simulink model "gm_lab3_p9"  (R2020a)
settings: Solver=VariableStepAuto  StartTime=0.0  StopTime=mp.test_signal.duration  RelTol=1e-3
InitFcn:
  | sm_callback_init
StopFcn:
  | sm_callback_stop
undefined symbols (not defined in the file or in its folder): mp
libraries: hdlsllib x10, simulink x3
(part 1 of 2)
settings Model: Creator=Owner  LastModifiedBy=Owner
settings DataIOCC: ReturnWorkspaceOutputs=off
settings OptimizationCC: BlockReduction=off  ConditionallyExecuteInputs=off  DefaultParameterBehavior=Inlined
settings DebuggingCC: AlgebraicLoopMsg=error  ArtificialAlgebraicLoopMsg=none  InheritedTsInSrcMsg=none
settings HardwareCC: ProdBitPerPointer=32  ProdBitPerSizeT=32  ProdBitPerPtrDiffT=32  ProdLargestAtomicFloat=None  ProdIntDivRoundTo=Undefined  ProdEndianess=Unspecified  ProdWordSize=32  ProdHWDeviceType=ASIC/FPGA->ASIC/FPGA  TargetBitPerPointer=64  TargetBitPerSizeT=64  TargetBitPerPtrDiffT=64  TargetLongLongMode=on  TargetIntDivRoundTo=Zero  TargetEndianess=LittleEndian  TargetWordSize=64  TargetHWDeviceType=Custom Processor->MATLAB Host Computer  ProdEqTarget=off

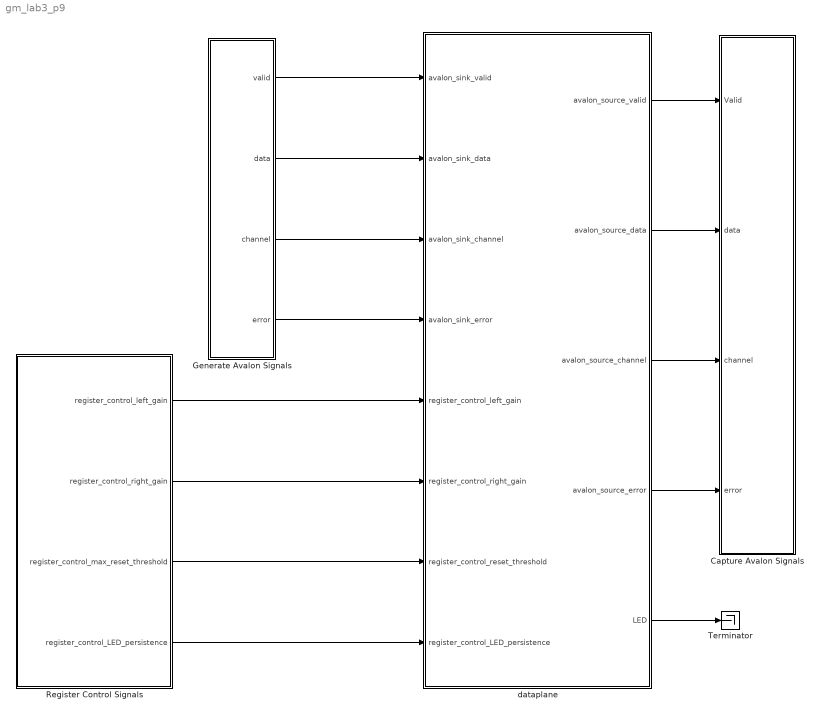
== system gm_lab3_p9 ==
  Capture Avalon Signals : Subsystem
  Generate Avalon Signals : Subsystem
  Register Control Signals : Subsystem
  Terminator : Terminator
  dataplane : Subsystem  TreatAsAtomicUnit=on
  wires:
  dataplane/5(LED) -> Terminator/1
  Register Control Signals/4(register_control_LED_persistence) -> dataplane/8(register_control_LED_persistence)
  Register Control Signals/3(register_control_max_reset_threshold) -> dataplane/7(register_control_reset_threshold)
  Register Control Signals/1(register_control_left_gain) -> dataplane/5(register_control_left_gain)
  Register Control Signals/2(register_control_right_gain) -> dataplane/6(register_control_right_gain)
  dataplane/4(avalon_source_error) -> Capture Avalon Signals/4(error)
  dataplane/3(avalon_source_channel) -> Capture Avalon Signals/3(channel)
  dataplane/2(avalon_source_data) -> Capture Avalon Signals/2(data)
  dataplane/1(avalon_source_valid) -> Capture Avalon Signals/1(Valid)
  Generate Avalon Signals/4(error) -> dataplane/4(avalon_sink_error)
  Generate Avalon Signals/3(channel) -> dataplane/3(avalon_sink_channel)
  Generate Avalon Signals/2(data) -> dataplane/2(avalon_sink_data)
  Generate Avalon Signals/1(valid) -> dataplane/1(avalon_sink_valid)

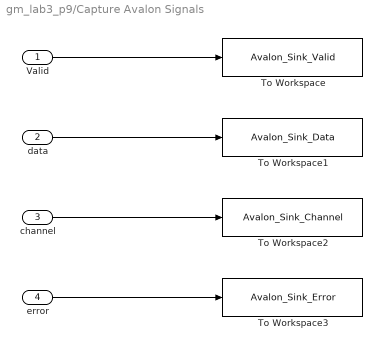
== system gm_lab3_p9/Capture Avalon Signals ==
  Valid : Inport
  data : Inport  Port=2
  channel : Inport  Port=3
  error : Inport  Port=4
  To Workspace : ToWorkspace  VariableName=Avalon_Sink_Valid  SampleTime=-1
      settings: Save2DSignal=2-D array (concatenate along first dimension)
  To Workspace1 : ToWorkspace  VariableName=Avalon_Sink_Data  SampleTime=-1
      settings: Save2DSignal=2-D array (concatenate along first dimension)
  To Workspace2 : ToWorkspace  VariableName=Avalon_Sink_Channel  SampleTime=-1
      settings: Save2DSignal=2-D array (concatenate along first dimension)
  To Workspace3 : ToWorkspace  VariableName=Avalon_Sink_Error  SampleTime=-1
      settings: Save2DSignal=2-D array (concatenate along first dimension)
  wires:
  error/1 -> To Workspace3/1
  channel/1 -> To Workspace2/1
  data/1 -> To Workspace1/1
  Valid/1 -> To Workspace/1

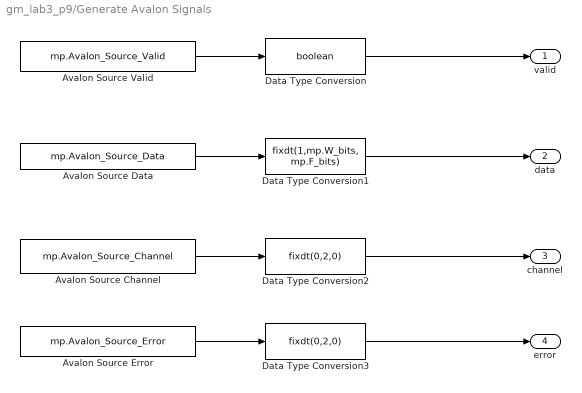
== system gm_lab3_p9/Generate Avalon Signals ==
  Avalon Source Channel : FromWorkspace  VariableName=mp.Avalon_Source_Channel  OutDataTypeStr=double  SampleTime=mp.Ts_system
  Avalon Source Data : FromWorkspace  VariableName=mp.Avalon_Source_Data  OutDataTypeStr=double  SampleTime=mp.Ts_system
  Avalon Source Error : FromWorkspace  VariableName=mp.Avalon_Source_Error  OutDataTypeStr=double  SampleTime=mp.Ts_system
  Avalon Source Valid : FromWorkspace  VariableName=mp.Avalon_Source_Valid  OutDataTypeStr=double  SampleTime=mp.Ts_system
  Data Type Conversion : DataTypeConversion  OutDataTypeStr=boolean  RndMeth=Nearest
  Data Type Conversion1 : DataTypeConversion  OutDataTypeStr=fixdt(1,mp.W_bits, mp.F_bits)  RndMeth=Nearest
  Data Type Conversion2 : DataTypeConversion  OutDataTypeStr=fixdt(0,2,0)  RndMeth=Nearest
  Data Type Conversion3 : DataTypeConversion  OutDataTypeStr=fixdt(0,2,0)  RndMeth=Nearest
  valid : Outport
  data : Outport  Port=2
  channel : Outport  Port=3
  error : Outport  Port=4
  wires:
  Avalon Source Error/1 -> Data Type Conversion3/1
  Data Type Conversion3/1 -> error/1
  Avalon Source Channel/1 -> Data Type Conversion2/1
  Data Type Conversion2/1 -> channel/1
  Data Type Conversion1/1 -> data/1
  Avalon Source Data/1 -> Data Type Conversion1/1
  Avalon Source Valid/1 -> Data Type Conversion/1
  Data Type Conversion/1 -> valid/1

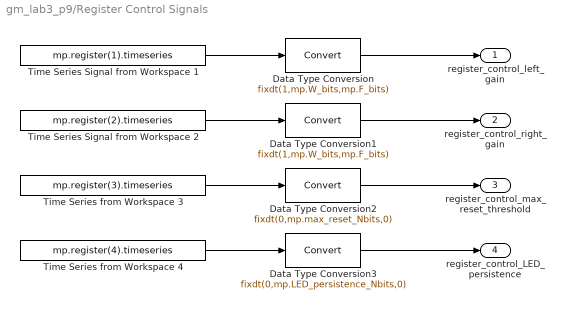
== system gm_lab3_p9/Register Control Signals ==
  Data Type Conversion : DataTypeConversion  OutDataTypeStr=fixdt(1,mp.W_bits,mp.F_bits)
  Data Type Conversion1 : DataTypeConversion  OutDataTypeStr=fixdt(1,mp.W_bits,mp.F_bits)
  Data Type Conversion2 : DataTypeConversion  OutDataTypeStr=fixdt(0,mp.max_reset_Nbits,0)
  Data Type Conversion3 : DataTypeConversion  OutDataTypeStr=fixdt(0,mp.LED_persistence_Nbits,0)
  Time Series Signal from Workspace 1 : FromWorkspace  VariableName=mp.register(1).timeseries  OutDataTypeStr=double  SampleTime=mp.Ts_system
  Time Series Signal from Workspace 2 : FromWorkspace  VariableName=mp.register(2).timeseries  OutDataTypeStr=double  SampleTime=mp.Ts_system
  Time Series from Workspace 3 : FromWorkspace  VariableName=mp.register(3).timeseries  OutDataTypeStr=double  SampleTime=mp.Ts_system
  Time Series from Workspace 4 : FromWorkspace  VariableName=mp.register(4).timeseries  OutDataTypeStr=double  SampleTime=mp.Ts_system
  register_control_left_gain : Outport
  register_control_right_gain : Outport  Port=2
  register_control_max_reset_threshold : Outport  Port=3
  register_control_LED_persistence : Outport  Port=4
  wires:
  Time Series from Workspace 3/1 -> Data Type Conversion2/1
  Time Series from Workspace 4/1 -> Data Type Conversion3/1
  Data Type Conversion3/1 -> register_control_LED_persistence/1
  Data Type Conversion2/1 -> register_control_max_reset_threshold/1
  Data Type Conversion1/1 -> register_control_right_gain/1
  Time Series Signal from Workspace 2/1 -> Data Type Conversion1/1
  Data Type Conversion/1 -> register_control_left_gain/1
  Time Series Signal from Workspace 1/1 -> Data Type Conversion/1

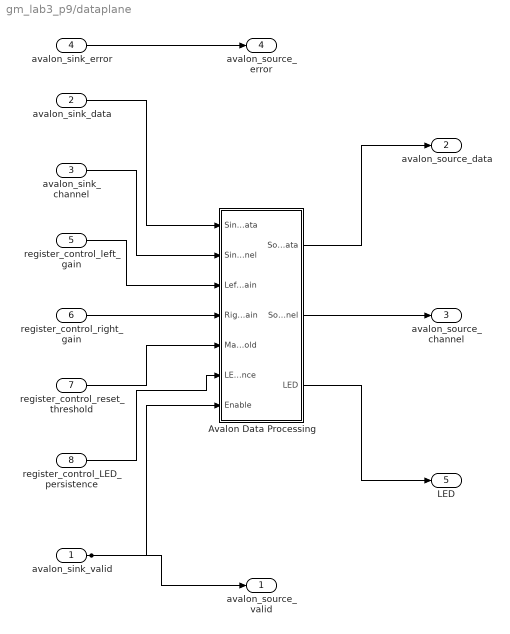
== system gm_lab3_p9/dataplane ==
  avalon_sink_valid : Inport  OutDataTypeStr=boolean  PortDimensions=1  SampleTime=1.01725260416667e-08
  avalon_sink_data : Inport  Port=2  OutDataTypeStr=fixdt(1, 32, 28)  PortDimensions=1  SampleTime=1.01725260416667e-08
  avalon_sink_channel : Inport  Port=3  OutDataTypeStr=fixdt(0, 2, 0)  PortDimensions=1  SampleTime=1.01725260416667e-08
  avalon_sink_error : Inport  Port=4  OutDataTypeStr=fixdt(0, 2, 0)  PortDimensions=1  SampleTime=1.01725260416667e-08
  register_control_left_gain : Inport  Port=5  OutDataTypeStr=fixdt(1, 32, 28)  PortDimensions=1  SampleTime=1.01725260416667e-08
  register_control_right_gain : Inport  Port=6  OutDataTypeStr=fixdt(1, 32, 28)  PortDimensions=1  SampleTime=1.01725260416667e-08
  register_control_reset_threshold : Inport  Port=7  OutDataTypeStr=fixdt(0, 18, 0)  PortDimensions=1  SampleTime=1.01725260416667e-08
  register_control_LED_persistence : Inport  Port=8  OutDataTypeStr=fixdt(0, 15, 0)  PortDimensions=1  SampleTime=1.01725260416667e-08
  Avalon Data Processing : Subsystem
  avalon_source_valid : Outport  VectorParamsAs1DForOutWhenUnconnected=off
  avalon_source_data : Outport  Port=2  VectorParamsAs1DForOutWhenUnconnected=off
  avalon_source_channel : Outport  Port=3  VectorParamsAs1DForOutWhenUnconnected=off
  avalon_source_error : Outport  Port=4  VectorParamsAs1DForOutWhenUnconnected=off
  LED : Outport  Port=5  VectorParamsAs1DForOutWhenUnconnected=off
  wires:
  avalon_sink_valid/1 -> avalon_source_valid/1, Avalon Data Processing/7(Enable)
  avalon_sink_data/1 -> Avalon Data Processing/1(Sink_Data)
  avalon_sink_channel/1 -> Avalon Data Processing/2(Sink_Channel)
  avalon_sink_error/1 -> avalon_source_error/1
  register_control_left_gain/1 -> Avalon Data Processing/3(Left_Gain)
  register_control_right_gain/1 -> Avalon Data Processing/4(Right_Gain)
  register_control_reset_threshold/1 -> Avalon Data Processing/5(Max_Reset_Threshold)
  register_control_LED_persistence/1 -> Avalon Data Processing/6(LED_persistence)
  Avalon Data Processing/1(Source_Data) -> avalon_source_data/1
  Avalon Data Processing/2(Source_Channel) -> avalon_source_channel/1
  Avalon Data Processing/3(LED) -> LED/1

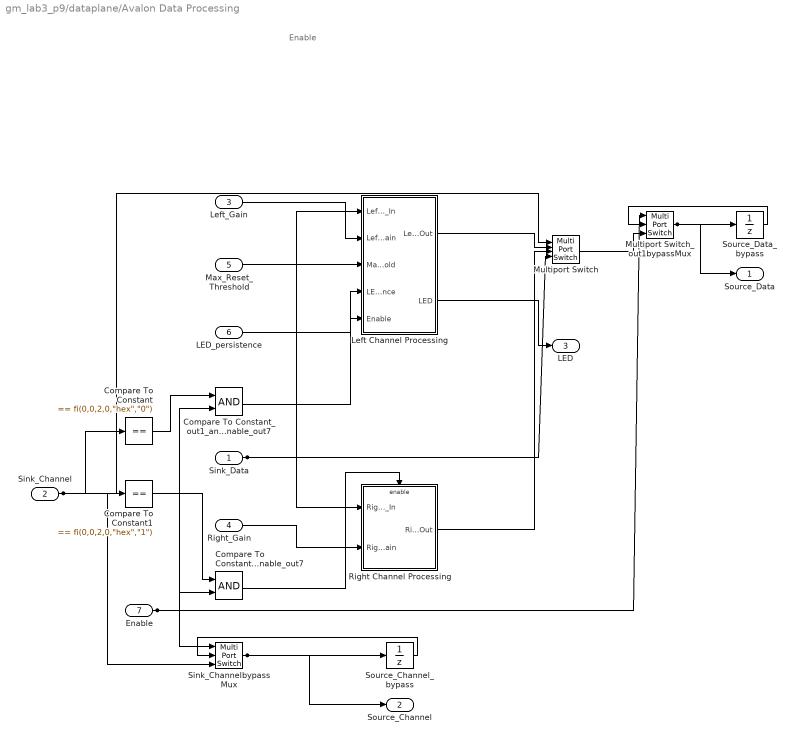
== system gm_lab3_p9/dataplane/Avalon Data Processing ==
  note: Enable
  Sink_Data : Inport  OutDataTypeStr=fixdt(1, 32, 28)  PortDimensions=1  SampleTime=1.01725260416667e-08
  Sink_Channel : Inport  Port=2  OutDataTypeStr=fixdt(0, 2, 0)  PortDimensions=1  SampleTime=1.01725260416667e-08
  Left_Gain : Inport  Port=3  OutDataTypeStr=fixdt(1, 32, 28)  PortDimensions=1  SampleTime=1.01725260416667e-08
  Right_Gain : Inport  Port=4  OutDataTypeStr=fixdt(1, 32, 28)  PortDimensions=1  SampleTime=1.01725260416667e-08
  Max_Reset_Threshold : Inport  Port=5  OutDataTypeStr=fixdt(0, 18, 0)  PortDimensions=1  SampleTime=1.01725260416667e-08
  LED_persistence : Inport  Port=6  OutDataTypeStr=fixdt(0, 15, 0)  PortDimensions=1  SampleTime=1.01725260416667e-08
  Enable : Inport  Port=7  OutDataTypeStr=boolean  SampleTime=1.01725260416667e-08
  Compare To Constant : simulink/Logic and Bit Operations/Compare To Constant  relop===  const="fi(0,0,2,0,\"hex\",\"0\")"  OutDataTypeStr=boolean
  Compare To Constant1 : simulink/Logic and Bit Operations/Compare To Constant  relop===  const="fi(0,0,2,0,\"hex\",\"1\")"  OutDataTypeStr=boolean
  Compare To Constant1_out1_and_Enable_out7 : Logic  AllPortsSameDT=off  OutDataTypeStr=boolean  SampleTime=1.01725260416667e-08
  Compare To Constant_out1_and_Enable_out7 : Logic  AllPortsSameDT=off  OutDataTypeStr=boolean  SampleTime=1.01725260416667e-08
  Left Channel Processing : Subsystem
  Multiport Switch : MultiPortSwitch  DataPortOrder=Zero-based contiguous  DiagnosticForDefault=None  zeroidx=on  OutDataTypeStr=fixdt(1, 32, 28)  SampleTime=1.01725260416667e-08
  Multiport Switch_out1bypassMux : MultiPortSwitch  DataPortOrder=Zero-based contiguous  Inputs=2  zeroidx=on  OutDataTypeStr=fixdt(1, 32, 28)  SampleTime=1.01725260416667e-08
  Right Channel Processing : Subsystem
  Sink_ChannelbypassMux : MultiPortSwitch  DataPortOrder=Zero-based contiguous  Inputs=2  zeroidx=on  OutDataTypeStr=fixdt(0, 2, 0)  SampleTime=1.01725260416667e-08
  Source_Channel_bypass : UnitDelay  SampleTime=1.01725260416667e-08
  Source_Data_bypass : UnitDelay  SampleTime=1.01725260416667e-08
  Source_Data : Outport  InitialOutput=0  VectorParamsAs1DForOutWhenUnconnected=off
  Source_Channel : Outport  Port=2  InitialOutput=0  VectorParamsAs1DForOutWhenUnconnected=off
  LED : Outport  Port=3  InitialOutput=0  VectorParamsAs1DForOutWhenUnconnected=off
  wires:
  Enable/1 -> Sink_ChannelbypassMux/1, Multiport Switch_out1bypassMux/1, Compare To Constant1_out1_and_Enable_out7/2, Compare To Constant_out1_and_Enable_out7/2
  Sink_Data/1 -> Multiport Switch/4, Right Channel Processing/1(Right_Data_In), Left Channel Processing/1(Left_Data_In)
  Sink_Channel/1 -> Multiport Switch/1, Compare To Constant1/1, Compare To Constant/1, Sink_ChannelbypassMux/3
  Left_Gain/1 -> Left Channel Processing/2(Left_Gain)
  Right_Gain/1 -> Right Channel Processing/2(Right_Gain)
  Max_Reset_Threshold/1 -> Left Channel Processing/3(Max_Reset_Threshold)
  LED_persistence/1 -> Left Channel Processing/4(LED_persistence)
  Compare To Constant/1 -> Compare To Constant_out1_and_Enable_out7/1
  Compare To Constant1/1 -> Compare To Constant1_out1_and_Enable_out7/1
  Left Channel Processing/1(Left_Data_Out) -> Multiport Switch/2
  Left Channel Processing/2(LED) -> LED/1
  Multiport Switch/1 -> Multiport Switch_out1bypassMux/3
  Right Channel Processing/1(Right_Data_Out) -> Multiport Switch/3
  Compare To Constant_out1_and_Enable_out7/1 -> Left Channel Processing/5(Enable)
  Compare To Constant1_out1_and_Enable_out7/1 -> Right Channel Processing/Enable
  Multiport Switch_out1bypassMux/1 -> Source_Data_bypass/1, Source_Data/1
  Source_Data_bypass/1 -> Multiport Switch_out1bypassMux/2
  Sink_ChannelbypassMux/1 -> Source_Channel_bypass/1, Source_Channel/1
  Source_Channel_bypass/1 -> Sink_ChannelbypassMux/2

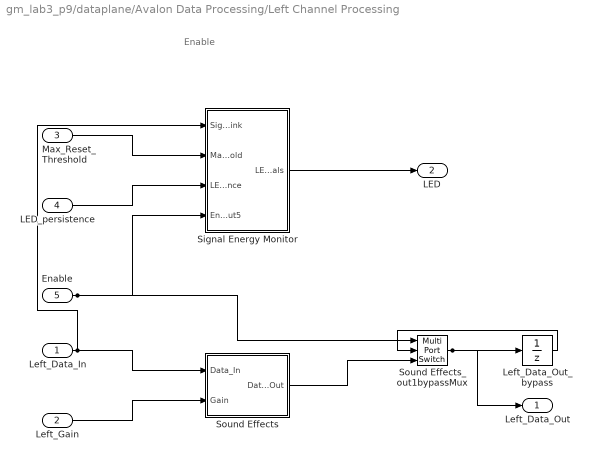
== system gm_lab3_p9/dataplane/Avalon Data Processing/Left Channel Processing ==
  note: Enable
  Left_Data_In : Inport  OutDataTypeStr=fixdt(1, 32, 28)  PortDimensions=1  SampleTime=1.01725260416667e-08
  Left_Gain : Inport  Port=2  OutDataTypeStr=fixdt(1, 32, 28)  PortDimensions=1  SampleTime=1.01725260416667e-08
  Max_Reset_Threshold : Inport  Port=3  OutDataTypeStr=fixdt(0, 18, 0)  PortDimensions=1  SampleTime=1.01725260416667e-08
  LED_persistence : Inport  Port=4  OutDataTypeStr=fixdt(0, 15, 0)  PortDimensions=1  SampleTime=1.01725260416667e-08
  Enable : Inport  Port=5  OutDataTypeStr=boolean  SampleTime=1.01725260416667e-08
  Left_Data_Out_bypass : UnitDelay  SampleTime=1.01725260416667e-08
  Signal Energy Monitor : Subsystem
  Sound Effects : Subsystem
  Sound Effects_out1bypassMux : MultiPortSwitch  DataPortOrder=Zero-based contiguous  Inputs=2  zeroidx=on  OutDataTypeStr=fixdt(1, 32, 28)  SampleTime=1.01725260416667e-08
  Left_Data_Out : Outport  InitialOutput=0  VectorParamsAs1DForOutWhenUnconnected=off
  LED : Outport  Port=2  InitialOutput=0  VectorParamsAs1DForOutWhenUnconnected=off
  wires:
  Enable/1 -> Sound Effects_out1bypassMux/1, Signal Energy Monitor/4(Enable_out5)
  Left_Data_In/1 -> Signal Energy Monitor/1(Signal_Sink), Sound Effects/1(Data_In)
  Left_Gain/1 -> Sound Effects/2(Gain)
  Max_Reset_Threshold/1 -> Signal Energy Monitor/2(Max_Reset_Threshold)
  LED_persistence/1 -> Signal Energy Monitor/3(LED_persistence)
  Signal Energy Monitor/1(LED_Signals) -> LED/1
  Sound Effects/1(Data_Out) -> Sound Effects_out1bypassMux/3
  Sound Effects_out1bypassMux/1 -> Left_Data_Out_bypass/1, Left_Data_Out/1
  Left_Data_Out_bypass/1 -> Sound Effects_out1bypassMux/2

== system gm_lab3_p9/dataplane/Avalon Data Processing/Right Channel Processing ==
  note: Enable
  Right_Data_In : Inport  OutDataTypeStr=fixdt(1, 32, 28)  PortDimensions=1  SampleTime=1.01725260416667e-08
  Right_Gain : Inport  Port=2  OutDataTypeStr=fixdt(1, 32, 28)  PortDimensions=1  SampleTime=1.01725260416667e-08
  Enable : EnablePort  OutDataTypeStr=boolean
  Sound Effects : Subsystem
  Right_Data_Out : Outport  InitialOutput=0  VectorParamsAs1DForOutWhenUnconnected=off
  wires:
  Right_Data_In/1 -> Sound Effects/1(Data_In)
  Right_Gain/1 -> Sound Effects/2(Gain)
  Sound Effects/1(Data_Out) -> Right_Data_Out/1

== system gm_lab3_p9/dataplane/Avalon Data Processing/Left Channel Processing/Signal Energy Monitor ==
  Signal_Sink : Inport  OutDataTypeStr=fixdt(1, 32, 28)  PortDimensions=1  SampleTime=1.01725260416667e-08
  Max_Reset_Threshold : Inport  Port=2  OutDataTypeStr=fixdt(0, 18, 0)  PortDimensions=1  SampleTime=1.01725260416667e-08
  LED_persistence : Inport  Port=3  OutDataTypeStr=fixdt(0, 15, 0)  PortDimensions=1  SampleTime=1.01725260416667e-08
  Enable_out5 : Inport  Port=4  OutDataTypeStr=boolean  SampleTime=1.01725260416667e-08
  LED_Driver : Subsystem
  Normalize Signal : Subsystem
  LED_Signals : Outport  InitialOutput=0  VectorParamsAs1DForOutWhenUnconnected=off
  wires:
  Signal_Sink/1 -> Normalize Signal/1(Signal_Sink)
  Max_Reset_Threshold/1 -> Normalize Signal/2(Max_Reset_Threshold)
  LED_persistence/1 -> LED_Driver/2(LED_persistence)
  LED_Driver/1(LED_Signals) -> LED_Signals/1
  Normalize Signal/1(Normalized_Signal_Energy) -> LED_Driver/1(Normalized_Signal)
  Enable_out5/1 -> Normalize Signal/3(Enable_out5), LED_Driver/3(Enable_out5)

== system gm_lab3_p9/dataplane/Avalon Data Processing/Left Channel Processing/Sound Effects ==
  Data_In : Inport  OutDataTypeStr=fixdt(1, 32, 28)  PortDimensions=1  SampleTime=1.01725260416667e-08
  Gain : Inport  Port=2  OutDataTypeStr=fixdt(1, 32, 28)  PortDimensions=1  SampleTime=1.01725260416667e-08
  Data Type Conversion : DataTypeConversion  OutDataTypeStr=fixdt(1, 32, 28)  RndMeth=Nearest  SampleTime=1.01725260416667e-08
  Product : Product  Inputs=**  OutDataTypeStr=fixdt(1, 64, 56)  SampleTime=1.01725260416667e-08
  Data_Out : Outport  InitialOutput=0
  wires:
  Data_In/1 -> Product/1
  Gain/1 -> Product/2
  Data Type Conversion/1 -> Data_Out/1
  Product/1 -> Data Type Conversion/1

== system gm_lab3_p9/dataplane/Avalon Data Processing/Right Channel Processing/Sound Effects ==
  Data_In : Inport  OutDataTypeStr=fixdt(1, 32, 28)  PortDimensions=1  SampleTime=1.01725260416667e-08
  Gain : Inport  Port=2  OutDataTypeStr=fixdt(1, 32, 28)  PortDimensions=1  SampleTime=1.01725260416667e-08
  Data Type Conversion : DataTypeConversion  OutDataTypeStr=fixdt(1, 32, 28)  RndMeth=Nearest  SampleTime=1.01725260416667e-08
  Product : Product  Inputs=**  OutDataTypeStr=fixdt(1, 64, 56)  SampleTime=1.01725260416667e-08
  Data_Out : Outport  InitialOutput=0
  wires:
  Data_In/1 -> Product/1
  Gain/1 -> Product/2
  Data Type Conversion/1 -> Data_Out/1
  Product/1 -> Data Type Conversion/1

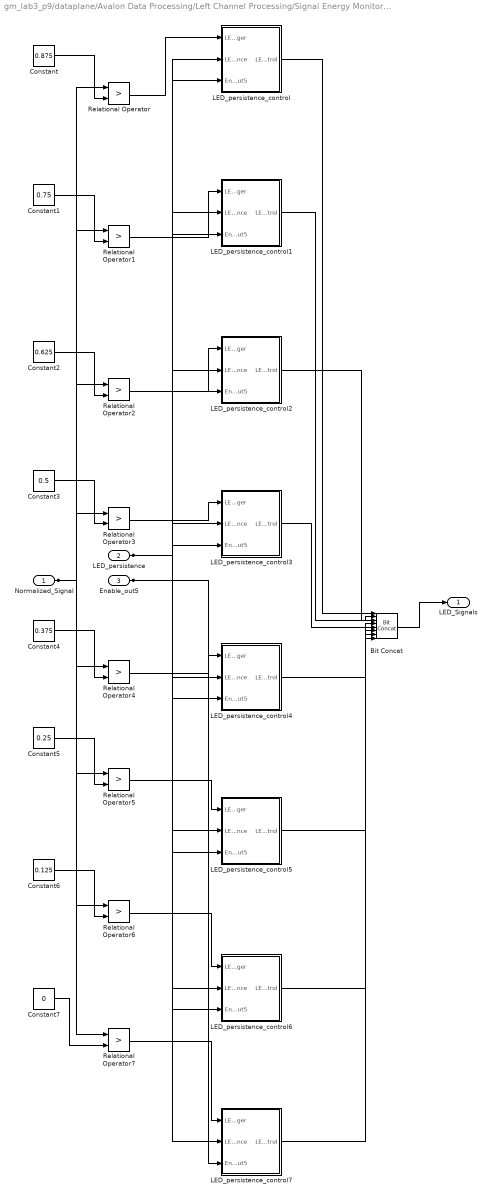
== system gm_lab3_p9/dataplane/Avalon Data Processing/Left Channel Processing/Signal Energy Monitor/LED_Driver ==
  Normalized_Signal : Inport  OutDataTypeStr=fixdt(1, 32, 28)  PortDimensions=1  SampleTime=1.01725260416667e-08
  LED_persistence : Inport  Port=2  OutDataTypeStr=fixdt(0, 15, 0)  PortDimensions=1  SampleTime=1.01725260416667e-08
  Enable_out5 : Inport  Port=3  OutDataTypeStr=boolean  SampleTime=1.01725260416667e-08
  Bit Concat : hdlsllib/Logic and Bit Operations/Bit Concat  numInputs=8
  Constant : Constant  Value=0.875  OutDataTypeStr=fixdt(1, 32, 28)  SampleTime=1.01725260416667e-08
  Constant1 : Constant  Value=0.75  OutDataTypeStr=fixdt(1, 32, 28)  SampleTime=1.01725260416667e-08
  Constant2 : Constant  Value=0.625  OutDataTypeStr=fixdt(1, 32, 28)  SampleTime=1.01725260416667e-08
  Constant3 : Constant  Value=0.5  OutDataTypeStr=fixdt(1, 32, 28)  SampleTime=1.01725260416667e-08
  Constant4 : Constant  Value=0.375  OutDataTypeStr=fixdt(1, 32, 28)  SampleTime=1.01725260416667e-08
  Constant5 : Constant  Value=0.25  OutDataTypeStr=fixdt(1, 32, 28)  SampleTime=1.01725260416667e-08
  Constant6 : Constant  Value=0.125  OutDataTypeStr=fixdt(1, 32, 28)  SampleTime=1.01725260416667e-08
  Constant7 : Constant  Value=0  OutDataTypeStr=fixdt(1, 32, 28)  SampleTime=1.01725260416667e-08
  LED_persistence_control : Subsystem
  LED_persistence_control1 : Subsystem
  LED_persistence_control2 : Subsystem
  LED_persistence_control3 : Subsystem
  LED_persistence_control4 : Subsystem
  LED_persistence_control5 : Subsystem
  LED_persistence_control6 : Subsystem
  LED_persistence_control7 : Subsystem
  Relational Operator{,1..7} (8 alike) : RelationalOperator  Operator=>  OutDataTypeStr=boolean  SampleTime=1.01725260416667e-08  RndMeth=Nearest
  LED_Signals : Outport  InitialOutput=0
  wires:
  Normalized_Signal/1 -> Relational Operator7/1, Relational Operator6/1, Relational Operator5/1, Relational Operator4/1, Relational Operator3/1, Relational Operator2/1, Relational Operator1/1, Relational Operator/1
  LED_persistence/1 -> LED_persistence_control7/2(LED_persistence), LED_persistence_control6/2(LED_persistence), LED_persistence_control5/2(LED_persistence), LED_persistence_control4/2(LED_persistence), LED_persistence_control3/2(LED_persistence), LED_persistence_control2/2(LED_persistence), LED_persistence_control1/2(LED_persistence), LED_persistence_control/2(LED_persistence)
  Bit Concat/1 -> LED_Signals/1
  Constant/1 -> Relational Operator/2
  Constant1/1 -> Relational Operator1/2
  Constant2/1 -> Relational Operator2/2
  Constant3/1 -> Relational Operator3/2
  Constant4/1 -> Relational Operator4/2
  Constant5/1 -> Relational Operator5/2
  Constant6/1 -> Relational Operator6/2
  Constant7/1 -> Relational Operator7/2
  LED_persistence_control/1(LED_control) -> Bit Concat/1
  LED_persistence_control1/1(LED_control) -> Bit Concat/2
  LED_persistence_control2/1(LED_control) -> Bit Concat/3
  LED_persistence_control3/1(LED_control) -> Bit Concat/4
  LED_persistence_control4/1(LED_control) -> Bit Concat/5
  LED_persistence_control5/1(LED_control) -> Bit Concat/6
  LED_persistence_control6/1(LED_control) -> Bit Concat/7
  LED_persistence_control7/1(LED_control) -> Bit Concat/8
  Relational Operator/1 -> LED_persistence_control/1(LED_trigger)
  Relational Operator1/1 -> LED_persistence_control1/1(LED_trigger)
  Relational Operator2/1 -> LED_persistence_control2/1(LED_trigger)
  Relational Operator3/1 -> LED_persistence_control3/1(LED_trigger)
  Relational Operator4/1 -> LED_persistence_control4/1(LED_trigger)
  Relational Operator5/1 -> LED_persistence_control5/1(LED_trigger)
  Relational Operator6/1 -> LED_persistence_control6/1(LED_trigger)
  Relational Operator7/1 -> LED_persistence_control7/1(LED_trigger)
  Enable_out5/1 -> LED_persistence_control7/3(Enable_out5), LED_persistence_control6/3(Enable_out5), LED_persistence_control5/3(Enable_out5), LED_persistence_control4/3(Enable_out5), LED_persistence_control3/3(Enable_out5), LED_persistence_control2/3(Enable_out5), LED_persistence_control1/3(Enable_out5), LED_persistence_control/3(Enable_out5)

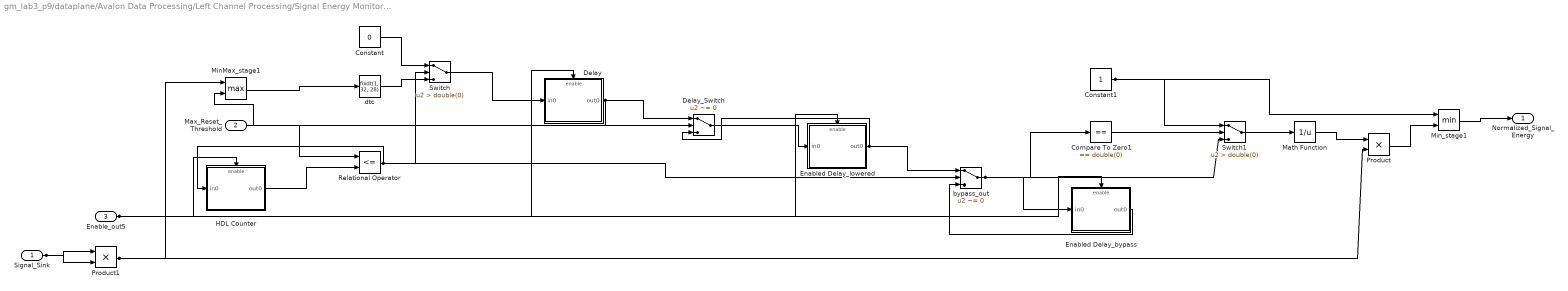
== system gm_lab3_p9/dataplane/Avalon Data Processing/Left Channel Processing/Signal Energy Monitor/Normalize Signal ==
  Signal_Sink : Inport  OutDataTypeStr=fixdt(1, 32, 28)  PortDimensions=1  SampleTime=1.01725260416667e-08
  Max_Reset_Threshold : Inport  Port=2  OutDataTypeStr=fixdt(0, 18, 0)  PortDimensions=1  SampleTime=1.01725260416667e-08
  Enable_out5 : Inport  Port=3  OutDataTypeStr=boolean  SampleTime=1.01725260416667e-08
  Compare To Zero1 : simulink/Logic and Bit Operations/Compare To Constant  relop===  const=double(0)  OutDataTypeStr=boolean
  Constant : Constant  Value=0  OutDataTypeStr=fixdt(1, 32, 28)  SampleTime=1.01725260416667e-08
  Constant1 : Constant  OutDataTypeStr=fixdt(1, 32, 28)  SampleTime=1.01725260416667e-08
  Delay : Subsystem
      settings: MinAlgLoopOccurrences=on
  Delay_Switch : Switch  Criteria=u2 ~= 0  Threshold=double(0)  OutDataTypeStr=fixdt(1, 32, 28)  SampleTime=1.01725260416667e-08
  Enabled Delay_bypass : Subsystem
      settings: MinAlgLoopOccurrences=on
  Enabled Delay_lowered : Subsystem
      settings: MinAlgLoopOccurrences=on
  HDL Counter : Subsystem
      settings: MinAlgLoopOccurrences=on
  Math Function : Math  Operator=reciprocal  OutDataTypeStr=fixdt(1,32,24)  RndMeth=Zero  SaturateOnIntegerOverflow=on
  MinMax_stage1 : MinMax  Function=max  Inputs=2
  Min_stage1 : MinMax  Inputs=2
  Product : Product  Inputs=**  OutDataTypeStr=fixdt(1, 32, 28)  SampleTime=1.01725260416667e-08
  Product1 : Product  Inputs=**  OutDataTypeStr=fixdt(1, 32, 28)  SampleTime=1.01725260416667e-08
  Relational Operator : RelationalOperator  Operator=<=  OutDataTypeStr=boolean  SampleTime=1.01725260416667e-08  RndMeth=Nearest
  Switch : Switch  Criteria=u2 > Threshold  Threshold=double(0)  OutDataTypeStr=fixdt(1, 32, 28)  SampleTime=1.01725260416667e-08
  Switch1 : Switch  Criteria=u2 > Threshold  Threshold=double(0)  OutDataTypeStr=fixdt(1, 32, 28)  SampleTime=1.01725260416667e-08
  bypass_out : Switch  Criteria=u2 ~= 0  Threshold=double(0)  OutDataTypeStr=fixdt(1, 32, 28)  SampleTime=1.01725260416667e-08
  dtc : DataTypeConversion  OutDataTypeStr=fixdt(1, 32, 28)  SampleTime=1.01725260416667e-08
  Normalized_Signal_Energy : Outport  InitialOutput=0
  wires:
  Signal_Sink/1 -> Product1/2, Product1/1
  Max_Reset_Threshold/1 -> Relational Operator/1
  Compare To Zero1/1 -> Switch1/2
  Constant/1 -> Switch/1
  Constant1/1 -> Switch1/1, Min_stage1/1
  Delay/1(out0) -> Delay_Switch/1, MinMax_stage1/2
  bypass_out/1 -> Switch1/3, Compare To Zero1/1, Enabled Delay_bypass/1(in0)
  HDL Counter/1(out0) -> Relational Operator/2
  Math Function/1 -> Product/1
  dtc/1 -> Switch/3
  Product/1 -> Min_stage1/2
  Product1/1 -> Product/2, MinMax_stage1/1
  Relational Operator/1 -> Switch/2, HDL Counter/1(in0), bypass_out/2, Delay_Switch/2
  Switch/1 -> Delay/1(in0)
  Switch1/1 -> Math Function/1
  Enabled Delay_lowered/1(out0) -> bypass_out/1, Delay_Switch/3
  Delay_Switch/1 -> Enabled Delay_lowered/1(in0)
  Enabled Delay_bypass/1(out0) -> bypass_out/3
  Enable_out5/1 -> Enabled Delay_bypass/Enable, Enabled Delay_lowered/Enable, HDL Counter/Enable, Delay/Enable
  Min_stage1/1 -> Normalized_Signal_Energy/1
  MinMax_stage1/1 -> dtc/1

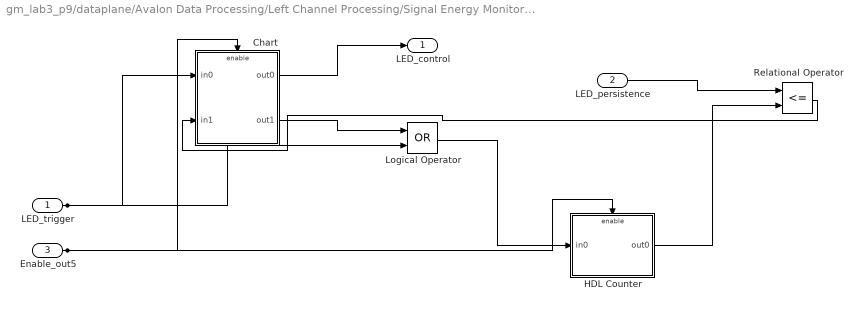
== system gm_lab3_p9/dataplane/Avalon Data Processing/Left Channel Processing/Signal Energy Monitor/LED_Driver/LED_persistence_control ==
  LED_trigger : Inport  OutDataTypeStr=boolean  PortDimensions=1  SampleTime=1.01725260416667e-08
  LED_persistence : Inport  Port=2  OutDataTypeStr=fixdt(0, 15, 0)  PortDimensions=1  SampleTime=1.01725260416667e-08
  Enable_out5 : Inport  Port=3  OutDataTypeStr=boolean  SampleTime=1.01725260416667e-08
  Chart : Subsystem
      settings: MinAlgLoopOccurrences=on
  HDL Counter : Subsystem
      settings: MinAlgLoopOccurrences=on
  Logical Operator : Logic  Operator=OR  AllPortsSameDT=off  OutDataTypeStr=boolean  SampleTime=1.01725260416667e-08
  Relational Operator : RelationalOperator  Operator=<=  OutDataTypeStr=boolean  SampleTime=1.01725260416667e-08  RndMeth=Nearest
  LED_control : Outport  InitialOutput=0
  wires:
  LED_trigger/1 -> Logical Operator/2, Chart/1(in0)
  LED_persistence/1 -> Relational Operator/1
  Chart/1(out0) -> LED_control/1
  Chart/2(out1) -> Logical Operator/1
  HDL Counter/1(out0) -> Relational Operator/2
  Logical Operator/1 -> HDL Counter/1(in0)
  Relational Operator/1 -> Chart/2(in1)
  Enable_out5/1 -> HDL Counter/Enable, Chart/Enable

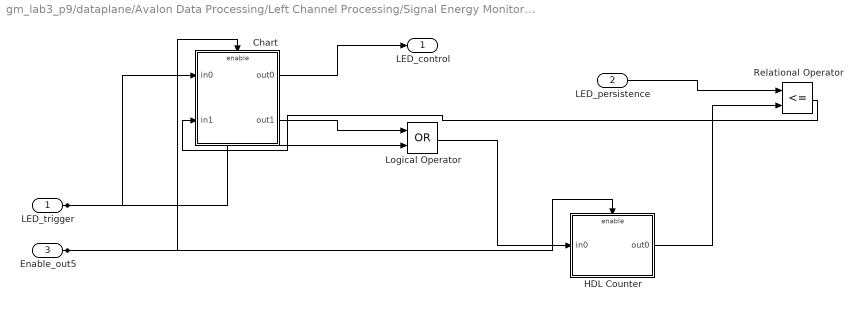
== system gm_lab3_p9/dataplane/Avalon Data Processing/Left Channel Processing/Signal Energy Monitor/LED_Driver/LED_persistence_control1 ==
  LED_trigger : Inport  OutDataTypeStr=boolean  PortDimensions=1  SampleTime=1.01725260416667e-08
  LED_persistence : Inport  Port=2  OutDataTypeStr=fixdt(0, 15, 0)  PortDimensions=1  SampleTime=1.01725260416667e-08
  Enable_out5 : Inport  Port=3  OutDataTypeStr=boolean  SampleTime=1.01725260416667e-08
  Chart : Subsystem
      settings: MinAlgLoopOccurrences=on
  HDL Counter : Subsystem
      settings: MinAlgLoopOccurrences=on
  Logical Operator : Logic  Operator=OR  AllPortsSameDT=off  OutDataTypeStr=boolean  SampleTime=1.01725260416667e-08
  Relational Operator : RelationalOperator  Operator=<=  OutDataTypeStr=boolean  SampleTime=1.01725260416667e-08  RndMeth=Nearest
  LED_control : Outport  InitialOutput=0
  wires:
  LED_trigger/1 -> Logical Operator/2, Chart/1(in0)
  LED_persistence/1 -> Relational Operator/1
  Chart/1(out0) -> LED_control/1
  Chart/2(out1) -> Logical Operator/1
  HDL Counter/1(out0) -> Relational Operator/2
  Logical Operator/1 -> HDL Counter/1(in0)
  Relational Operator/1 -> Chart/2(in1)
  Enable_out5/1 -> HDL Counter/Enable, Chart/Enable

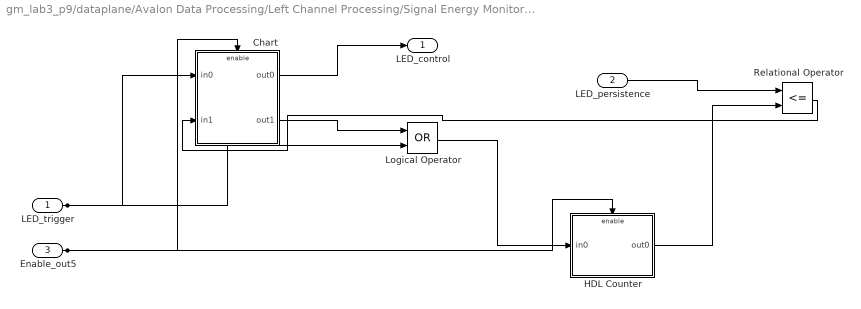
== system gm_lab3_p9/dataplane/Avalon Data Processing/Left Channel Processing/Signal Energy Monitor/LED_Driver/LED_persistence_control2 ==
  LED_trigger : Inport  OutDataTypeStr=boolean  PortDimensions=1  SampleTime=1.01725260416667e-08
  LED_persistence : Inport  Port=2  OutDataTypeStr=fixdt(0, 15, 0)  PortDimensions=1  SampleTime=1.01725260416667e-08
  Enable_out5 : Inport  Port=3  OutDataTypeStr=boolean  SampleTime=1.01725260416667e-08
  Chart : Subsystem
      settings: MinAlgLoopOccurrences=on
  HDL Counter : Subsystem
      settings: MinAlgLoopOccurrences=on
  Logical Operator : Logic  Operator=OR  AllPortsSameDT=off  OutDataTypeStr=boolean  SampleTime=1.01725260416667e-08
  Relational Operator : RelationalOperator  Operator=<=  OutDataTypeStr=boolean  SampleTime=1.01725260416667e-08  RndMeth=Nearest
  LED_control : Outport  InitialOutput=0
  wires:
  LED_trigger/1 -> Logical Operator/2, Chart/1(in0)
  LED_persistence/1 -> Relational Operator/1
  Chart/1(out0) -> LED_control/1
  Chart/2(out1) -> Logical Operator/1
  HDL Counter/1(out0) -> Relational Operator/2
  Logical Operator/1 -> HDL Counter/1(in0)
  Relational Operator/1 -> Chart/2(in1)
  Enable_out5/1 -> HDL Counter/Enable, Chart/Enable

== system gm_lab3_p9/dataplane/Avalon Data Processing/Left Channel Processing/Signal Energy Monitor/LED_Driver/LED_persistence_control3 ==
  LED_trigger : Inport  OutDataTypeStr=boolean  PortDimensions=1  SampleTime=1.01725260416667e-08
  LED_persistence : Inport  Port=2  OutDataTypeStr=fixdt(0, 15, 0)  PortDimensions=1  SampleTime=1.01725260416667e-08
  Enable_out5 : Inport  Port=3  OutDataTypeStr=boolean  SampleTime=1.01725260416667e-08
  Chart : Subsystem
      settings: MinAlgLoopOccurrences=on
  HDL Counter : Subsystem
      settings: MinAlgLoopOccurrences=on
  Logical Operator : Logic  Operator=OR  AllPortsSameDT=off  OutDataTypeStr=boolean  SampleTime=1.01725260416667e-08
  Relational Operator : RelationalOperator  Operator=<=  OutDataTypeStr=boolean  SampleTime=1.01725260416667e-08  RndMeth=Nearest
  LED_control : Outport  InitialOutput=0
  wires:
  LED_trigger/1 -> Logical Operator/2, Chart/1(in0)
  LED_persistence/1 -> Relational Operator/1
  Chart/1(out0) -> LED_control/1
  Chart/2(out1) -> Logical Operator/1
  HDL Counter/1(out0) -> Relational Operator/2
  Logical Operator/1 -> HDL Counter/1(in0)
  Relational Operator/1 -> Chart/2(in1)
  Enable_out5/1 -> HDL Counter/Enable, Chart/Enable

== system gm_lab3_p9/dataplane/Avalon Data Processing/Left Channel Processing/Signal Energy Monitor/LED_Driver/LED_persistence_control4 ==
  LED_trigger : Inport  OutDataTypeStr=boolean  PortDimensions=1  SampleTime=1.01725260416667e-08
  LED_persistence : Inport  Port=2  OutDataTypeStr=fixdt(0, 15, 0)  PortDimensions=1  SampleTime=1.01725260416667e-08
  Enable_out5 : Inport  Port=3  OutDataTypeStr=boolean  SampleTime=1.01725260416667e-08
  Chart : Subsystem
      settings: MinAlgLoopOccurrences=on
  HDL Counter : Subsystem
      settings: MinAlgLoopOccurrences=on
  Logical Operator : Logic  Operator=OR  AllPortsSameDT=off  OutDataTypeStr=boolean  SampleTime=1.01725260416667e-08
  Relational Operator : RelationalOperator  Operator=<=  OutDataTypeStr=boolean  SampleTime=1.01725260416667e-08  RndMeth=Nearest
  LED_control : Outport  InitialOutput=0
  wires:
  LED_trigger/1 -> Logical Operator/2, Chart/1(in0)
  LED_persistence/1 -> Relational Operator/1
  Chart/1(out0) -> LED_control/1
  Chart/2(out1) -> Logical Operator/1
  HDL Counter/1(out0) -> Relational Operator/2
  Logical Operator/1 -> HDL Counter/1(in0)
  Relational Operator/1 -> Chart/2(in1)
  Enable_out5/1 -> HDL Counter/Enable, Chart/Enable

== system gm_lab3_p9/dataplane/Avalon Data Processing/Left Channel Processing/Signal Energy Monitor/LED_Driver/LED_persistence_control5 ==
  LED_trigger : Inport  OutDataTypeStr=boolean  PortDimensions=1  SampleTime=1.01725260416667e-08
  LED_persistence : Inport  Port=2  OutDataTypeStr=fixdt(0, 15, 0)  PortDimensions=1  SampleTime=1.01725260416667e-08
  Enable_out5 : Inport  Port=3  OutDataTypeStr=boolean  SampleTime=1.01725260416667e-08
  Chart : Subsystem
      settings: MinAlgLoopOccurrences=on
  HDL Counter : Subsystem
      settings: MinAlgLoopOccurrences=on
  Logical Operator : Logic  Operator=OR  AllPortsSameDT=off  OutDataTypeStr=boolean  SampleTime=1.01725260416667e-08
  Relational Operator : RelationalOperator  Operator=<=  OutDataTypeStr=boolean  SampleTime=1.01725260416667e-08  RndMeth=Nearest
  LED_control : Outport  InitialOutput=0
  wires:
  LED_trigger/1 -> Logical Operator/2, Chart/1(in0)
  LED_persistence/1 -> Relational Operator/1
  Chart/1(out0) -> LED_control/1
  Chart/2(out1) -> Logical Operator/1
  HDL Counter/1(out0) -> Relational Operator/2
  Logical Operator/1 -> HDL Counter/1(in0)
  Relational Operator/1 -> Chart/2(in1)
  Enable_out5/1 -> HDL Counter/Enable, Chart/Enable

== system gm_lab3_p9/dataplane/Avalon Data Processing/Left Channel Processing/Signal Energy Monitor/LED_Driver/LED_persistence_control6 ==
  LED_trigger : Inport  OutDataTypeStr=boolean  PortDimensions=1  SampleTime=1.01725260416667e-08
  LED_persistence : Inport  Port=2  OutDataTypeStr=fixdt(0, 15, 0)  PortDimensions=1  SampleTime=1.01725260416667e-08
  Enable_out5 : Inport  Port=3  OutDataTypeStr=boolean  SampleTime=1.01725260416667e-08
  Chart : Subsystem
      settings: MinAlgLoopOccurrences=on
  HDL Counter : Subsystem
      settings: MinAlgLoopOccurrences=on
  Logical Operator : Logic  Operator=OR  AllPortsSameDT=off  OutDataTypeStr=boolean  SampleTime=1.01725260416667e-08
  Relational Operator : RelationalOperator  Operator=<=  OutDataTypeStr=boolean  SampleTime=1.01725260416667e-08  RndMeth=Nearest
  LED_control : Outport  InitialOutput=0
  wires:
  LED_trigger/1 -> Logical Operator/2, Chart/1(in0)
  LED_persistence/1 -> Relational Operator/1
  Chart/1(out0) -> LED_control/1
  Chart/2(out1) -> Logical Operator/1
  HDL Counter/1(out0) -> Relational Operator/2
  Logical Operator/1 -> HDL Counter/1(in0)
  Relational Operator/1 -> Chart/2(in1)
  Enable_out5/1 -> HDL Counter/Enable, Chart/Enable

== system gm_lab3_p9/dataplane/Avalon Data Processing/Left Channel Processing/Signal Energy Monitor/LED_Driver/LED_persistence_control7 ==
  LED_trigger : Inport  OutDataTypeStr=boolean  PortDimensions=1  SampleTime=1.01725260416667e-08
  LED_persistence : Inport  Port=2  OutDataTypeStr=fixdt(0, 15, 0)  PortDimensions=1  SampleTime=1.01725260416667e-08
  Enable_out5 : Inport  Port=3  OutDataTypeStr=boolean  SampleTime=1.01725260416667e-08
  Chart : Subsystem
      settings: MinAlgLoopOccurrences=on
  HDL Counter : Subsystem
      settings: MinAlgLoopOccurrences=on
  Logical Operator : Logic  Operator=OR  AllPortsSameDT=off  OutDataTypeStr=boolean  SampleTime=1.01725260416667e-08
  Relational Operator : RelationalOperator  Operator=<=  OutDataTypeStr=boolean  SampleTime=1.01725260416667e-08  RndMeth=Nearest
  LED_control : Outport  InitialOutput=0
  wires:
  LED_trigger/1 -> Logical Operator/2, Chart/1(in0)
  LED_persistence/1 -> Relational Operator/1
  Chart/1(out0) -> LED_control/1
  Chart/2(out1) -> Logical Operator/1
  HDL Counter/1(out0) -> Relational Operator/2
  Logical Operator/1 -> HDL Counter/1(in0)
  Relational Operator/1 -> Chart/2(in1)
  Enable_out5/1 -> HDL Counter/Enable, Chart/Enable

== system gm_lab3_p9/dataplane/Avalon Data Processing/Left Channel Processing/Signal Energy Monitor/Normalize Signal/Delay ==
  in0 : Inport  OutDataTypeStr=fixdt(1, 32, 28)  SampleTime=1.01725260416667e-08
  Enable_out5 : EnablePort  OutDataTypeStr=boolean
  Delay : Delay  DelayLength=double(1)  InitialCondition=0
  out0 : Outport  OutDataTypeStr=fixdt(1, 32, 28)  InitialOutput=0
  wires:
  Delay/1 -> out0/1
  in0/1 -> Delay/1

== system gm_lab3_p9/dataplane/Avalon Data Processing/Left Channel Processing/Signal Energy Monitor/Normalize Signal/Enabled Delay_bypass ==
  in0 : Inport  OutDataTypeStr=fixdt(1, 32, 28)  SampleTime=1.01725260416667e-08
  Enable_out5 : EnablePort  OutDataTypeStr=boolean
  Enabled Delay_bypass : Delay  DelayLength=double(1)
  out0 : Outport  OutDataTypeStr=fixdt(1, 32, 28)  InitialOutput=0
  wires:
  Enabled Delay_bypass/1 -> out0/1
  in0/1 -> Enabled Delay_bypass/1

== system gm_lab3_p9/dataplane/Avalon Data Processing/Left Channel Processing/Signal Energy Monitor/Normalize Signal/Enabled Delay_lowered ==
  in0 : Inport  OutDataTypeStr=fixdt(1, 32, 28)  SampleTime=1.01725260416667e-08
  Enable_out5 : EnablePort  OutDataTypeStr=boolean
  Enabled Delay_lowered : Delay  DelayLength=double(1)  InitialCondition=0
  out0 : Outport  OutDataTypeStr=fixdt(1, 32, 28)  InitialOutput=0
  wires:
  Enabled Delay_lowered/1 -> out0/1
  in0/1 -> Enabled Delay_lowered/1

== system gm_lab3_p9/dataplane/Avalon Data Processing/Left Channel Processing/Signal Energy Monitor/Normalize Signal/HDL Counter ==
  in0 : Inport  OutDataTypeStr=boolean  SampleTime=1.01725260416667e-08
  Enable_out5 : EnablePort  OutDataTypeStr=boolean
  HDL Counter : hdlsllib/Sources/HDL Counter  CountType=Free running  CountInit=double(0)  CountStep=double(1)  CountMax=25  CountFromType=Initial value  CountFrom=double(0)  CountResetPort=on  CountLoadPort=off  CountEnbPort=off  CountDirPort=off  CountDataType=Unsigned  CountWordLen=18  CountFracLen=0  CountSampTime=1.01725260416667e-08
  out0 : Outport  OutDataTypeStr=fixdt(0, 18, 0)  InitialOutput=0
  wires:
  HDL Counter/1 -> out0/1
  in0/1 -> HDL Counter/1

== system gm_lab3_p9/dataplane/Avalon Data Processing/Left Channel Processing/Signal Energy Monitor/LED_Driver/LED_persistence_control/Chart ==
  in0 : Inport  OutDataTypeStr=boolean  SampleTime=1.01725260416667e-08
  in1 : Inport  Port=2  OutDataTypeStr=boolean  SampleTime=1.01725260416667e-08
  Enable_out5 : EnablePort  OutDataTypeStr=boolean
  Chart : Subsystem
  out0 : Outport  OutDataTypeStr=boolean  InitialOutput=0
  out1 : Outport  Port=2  OutDataTypeStr=boolean  InitialOutput=0
  wires:
  Chart/1(LED_signal) -> out0/1
  Chart/2(counter_reset) -> out1/1
  in0/1 -> Chart/1(LED_trigger)
  in1/1 -> Chart/2(count_reached)

== system gm_lab3_p9/dataplane/Avalon Data Processing/Left Channel Processing/Signal Energy Monitor/LED_Driver/LED_persistence_control/HDL Counter ==
  in0 : Inport  OutDataTypeStr=boolean  SampleTime=1.01725260416667e-08
  Enable_out5 : EnablePort  OutDataTypeStr=boolean
  HDL Counter : hdlsllib/Sources/HDL Counter  CountType=Free running  CountInit=double(0)  CountStep=double(1)  CountMax=25  CountFromType=Initial value  CountFrom=double(0)  CountResetPort=on  CountLoadPort=off  CountEnbPort=off  CountDirPort=off  CountDataType=Unsigned  CountWordLen=15  CountFracLen=0  CountSampTime=1.01725260416667e-08
  out0 : Outport  OutDataTypeStr=fixdt(0, 15, 0)  InitialOutput=0
  wires:
  HDL Counter/1 -> out0/1
  in0/1 -> HDL Counter/1

== system gm_lab3_p9/dataplane/Avalon Data Processing/Left Channel Processing/Signal Energy Monitor/LED_Driver/LED_persistence_control1/Chart ==
  in0 : Inport  OutDataTypeStr=boolean  SampleTime=1.01725260416667e-08
  in1 : Inport  Port=2  OutDataTypeStr=boolean  SampleTime=1.01725260416667e-08
  Enable_out5 : EnablePort  OutDataTypeStr=boolean
  Chart : Subsystem
  out0 : Outport  OutDataTypeStr=boolean  InitialOutput=0
  out1 : Outport  Port=2  OutDataTypeStr=boolean  InitialOutput=0
  wires:
  Chart/1(LED_signal) -> out0/1
  Chart/2(counter_reset) -> out1/1
  in0/1 -> Chart/1(LED_trigger)
  in1/1 -> Chart/2(count_reached)

== system gm_lab3_p9/dataplane/Avalon Data Processing/Left Channel Processing/Signal Energy Monitor/LED_Driver/LED_persistence_control1/HDL Counter ==
  in0 : Inport  OutDataTypeStr=boolean  SampleTime=1.01725260416667e-08
  Enable_out5 : EnablePort  OutDataTypeStr=boolean
  HDL Counter : hdlsllib/Sources/HDL Counter  CountType=Free running  CountInit=double(0)  CountStep=double(1)  CountMax=25  CountFromType=Initial value  CountFrom=double(0)  CountResetPort=on  CountLoadPort=off  CountEnbPort=off  CountDirPort=off  CountDataType=Unsigned  CountWordLen=15  CountFracLen=0  CountSampTime=1.01725260416667e-08
  out0 : Outport  OutDataTypeStr=fixdt(0, 15, 0)  InitialOutput=0
  wires:
  HDL Counter/1 -> out0/1
  in0/1 -> HDL Counter/1

== system gm_lab3_p9/dataplane/Avalon Data Processing/Left Channel Processing/Signal Energy Monitor/LED_Driver/LED_persistence_control2/Chart ==
  in0 : Inport  OutDataTypeStr=boolean  SampleTime=1.01725260416667e-08
  in1 : Inport  Port=2  OutDataTypeStr=boolean  SampleTime=1.01725260416667e-08
  Enable_out5 : EnablePort  OutDataTypeStr=boolean
  Chart : Subsystem
  out0 : Outport  OutDataTypeStr=boolean  InitialOutput=0
  out1 : Outport  Port=2  OutDataTypeStr=boolean  InitialOutput=0
  wires:
  Chart/1(LED_signal) -> out0/1
  Chart/2(counter_reset) -> out1/1
  in0/1 -> Chart/1(LED_trigger)
  in1/1 -> Chart/2(count_reached)

== system gm_lab3_p9/dataplane/Avalon Data Processing/Left Channel Processing/Signal Energy Monitor/LED_Driver/LED_persistence_control2/HDL Counter ==
  in0 : Inport  OutDataTypeStr=boolean  SampleTime=1.01725260416667e-08
  Enable_out5 : EnablePort  OutDataTypeStr=boolean
  HDL Counter : hdlsllib/Sources/HDL Counter  CountType=Free running  CountInit=double(0)  CountStep=double(1)  CountMax=25  CountFromType=Initial value  CountFrom=double(0)  CountResetPort=on  CountLoadPort=off  CountEnbPort=off  CountDirPort=off  CountDataType=Unsigned  CountWordLen=15  CountFracLen=0  CountSampTime=1.01725260416667e-08
  out0 : Outport  OutDataTypeStr=fixdt(0, 15, 0)  InitialOutput=0
  wires:
  HDL Counter/1 -> out0/1
  in0/1 -> HDL Counter/1

== system gm_lab3_p9/dataplane/Avalon Data Processing/Left Channel Processing/Signal Energy Monitor/LED_Driver/LED_persistence_control3/Chart ==
  in0 : Inport  OutDataTypeStr=boolean  SampleTime=1.01725260416667e-08
  in1 : Inport  Port=2  OutDataTypeStr=boolean  SampleTime=1.01725260416667e-08
  Enable_out5 : EnablePort  OutDataTypeStr=boolean
  Chart : Subsystem
  out0 : Outport  OutDataTypeStr=boolean  InitialOutput=0
  out1 : Outport  Port=2  OutDataTypeStr=boolean  InitialOutput=0
  wires:
  Chart/1(LED_signal) -> out0/1
  Chart/2(counter_reset) -> out1/1
  in0/1 -> Chart/1(LED_trigger)
  in1/1 -> Chart/2(count_reached)

== system gm_lab3_p9/dataplane/Avalon Data Processing/Left Channel Processing/Signal Energy Monitor/LED_Driver/LED_persistence_control3/HDL Counter ==
  in0 : Inport  OutDataTypeStr=boolean  SampleTime=1.01725260416667e-08
  Enable_out5 : EnablePort  OutDataTypeStr=boolean
  HDL Counter : hdlsllib/Sources/HDL Counter  CountType=Free running  CountInit=double(0)  CountStep=double(1)  CountMax=25  CountFromType=Initial value  CountFrom=double(0)  CountResetPort=on  CountLoadPort=off  CountEnbPort=off  CountDirPort=off  CountDataType=Unsigned  CountWordLen=15  CountFracLen=0  CountSampTime=1.01725260416667e-08
  out0 : Outport  OutDataTypeStr=fixdt(0, 15, 0)  InitialOutput=0
  wires:
  HDL Counter/1 -> out0/1
  in0/1 -> HDL Counter/1

== system gm_lab3_p9/dataplane/Avalon Data Processing/Left Channel Processing/Signal Energy Monitor/LED_Driver/LED_persistence_control4/Chart ==
  in0 : Inport  OutDataTypeStr=boolean  SampleTime=1.01725260416667e-08
  in1 : Inport  Port=2  OutDataTypeStr=boolean  SampleTime=1.01725260416667e-08
  Enable_out5 : EnablePort  OutDataTypeStr=boolean
  Chart : Subsystem
  out0 : Outport  OutDataTypeStr=boolean  InitialOutput=0
  out1 : Outport  Port=2  OutDataTypeStr=boolean  InitialOutput=0
  wires:
  Chart/1(LED_signal) -> out0/1
  Chart/2(counter_reset) -> out1/1
  in0/1 -> Chart/1(LED_trigger)
  in1/1 -> Chart/2(count_reached)

== system gm_lab3_p9/dataplane/Avalon Data Processing/Left Channel Processing/Signal Energy Monitor/LED_Driver/LED_persistence_control4/HDL Counter ==
  in0 : Inport  OutDataTypeStr=boolean  SampleTime=1.01725260416667e-08
  Enable_out5 : EnablePort  OutDataTypeStr=boolean
  HDL Counter : hdlsllib/Sources/HDL Counter  CountType=Free running  CountInit=double(0)  CountStep=double(1)  CountMax=25  CountFromType=Initial value  CountFrom=double(0)  CountResetPort=on  CountLoadPort=off  CountEnbPort=off  CountDirPort=off  CountDataType=Unsigned  CountWordLen=15  CountFracLen=0  CountSampTime=1.01725260416667e-08
  out0 : Outport  OutDataTypeStr=fixdt(0, 15, 0)  InitialOutput=0
  wires:
  HDL Counter/1 -> out0/1
  in0/1 -> HDL Counter/1

== system gm_lab3_p9/dataplane/Avalon Data Processing/Left Channel Processing/Signal Energy Monitor/LED_Driver/LED_persistence_control5/Chart ==
  in0 : Inport  OutDataTypeStr=boolean  SampleTime=1.01725260416667e-08
  in1 : Inport  Port=2  OutDataTypeStr=boolean  SampleTime=1.01725260416667e-08
  Enable_out5 : EnablePort  OutDataTypeStr=boolean
  Chart : Subsystem
  out0 : Outport  OutDataTypeStr=boolean  InitialOutput=0
  out1 : Outport  Port=2  OutDataTypeStr=boolean  InitialOutput=0
  wires:
  Chart/1(LED_signal) -> out0/1
  Chart/2(counter_reset) -> out1/1
  in0/1 -> Chart/1(LED_trigger)
  in1/1 -> Chart/2(count_reached)

== system gm_lab3_p9/dataplane/Avalon Data Processing/Left Channel Processing/Signal Energy Monitor/LED_Driver/LED_persistence_control5/HDL Counter ==
  in0 : Inport  OutDataTypeStr=boolean  SampleTime=1.01725260416667e-08
  Enable_out5 : EnablePort  OutDataTypeStr=boolean
  HDL Counter : hdlsllib/Sources/HDL Counter  CountType=Free running  CountInit=double(0)  CountStep=double(1)  CountMax=25  CountFromType=Initial value  CountFrom=double(0)  CountResetPort=on  CountLoadPort=off  CountEnbPort=off  CountDirPort=off  CountDataType=Unsigned  CountWordLen=15  CountFracLen=0  CountSampTime=1.01725260416667e-08
  out0 : Outport  OutDataTypeStr=fixdt(0, 15, 0)  InitialOutput=0
  wires:
  HDL Counter/1 -> out0/1
  in0/1 -> HDL Counter/1

== system gm_lab3_p9/dataplane/Avalon Data Processing/Left Channel Processing/Signal Energy Monitor/LED_Driver/LED_persistence_control6/Chart ==
  in0 : Inport  OutDataTypeStr=boolean  SampleTime=1.01725260416667e-08
  in1 : Inport  Port=2  OutDataTypeStr=boolean  SampleTime=1.01725260416667e-08
  Enable_out5 : EnablePort  OutDataTypeStr=boolean
  Chart : Subsystem
  out0 : Outport  OutDataTypeStr=boolean  InitialOutput=0
  out1 : Outport  Port=2  OutDataTypeStr=boolean  InitialOutput=0
  wires:
  Chart/1(LED_signal) -> out0/1
  Chart/2(counter_reset) -> out1/1
  in0/1 -> Chart/1(LED_trigger)
  in1/1 -> Chart/2(count_reached)

== system gm_lab3_p9/dataplane/Avalon Data Processing/Left Channel Processing/Signal Energy Monitor/LED_Driver/LED_persistence_control6/HDL Counter ==
  in0 : Inport  OutDataTypeStr=boolean  SampleTime=1.01725260416667e-08
  Enable_out5 : EnablePort  OutDataTypeStr=boolean
  HDL Counter : hdlsllib/Sources/HDL Counter  CountType=Free running  CountInit=double(0)  CountStep=double(1)  CountMax=25  CountFromType=Initial value  CountFrom=double(0)  CountResetPort=on  CountLoadPort=off  CountEnbPort=off  CountDirPort=off  CountDataType=Unsigned  CountWordLen=15  CountFracLen=0  CountSampTime=1.01725260416667e-08
  out0 : Outport  OutDataTypeStr=fixdt(0, 15, 0)  InitialOutput=0
  wires:
  HDL Counter/1 -> out0/1
  in0/1 -> HDL Counter/1

== system gm_lab3_p9/dataplane/Avalon Data Processing/Left Channel Processing/Signal Energy Monitor/LED_Driver/LED_persistence_control7/Chart ==
  in0 : Inport  OutDataTypeStr=boolean  SampleTime=1.01725260416667e-08
  in1 : Inport  Port=2  OutDataTypeStr=boolean  SampleTime=1.01725260416667e-08
  Enable_out5 : EnablePort  OutDataTypeStr=boolean
  Chart : Subsystem
  out0 : Outport  OutDataTypeStr=boolean  InitialOutput=0
  out1 : Outport  Port=2  OutDataTypeStr=boolean  InitialOutput=0
  wires:
  Chart/1(LED_signal) -> out0/1
  Chart/2(counter_reset) -> out1/1
  in0/1 -> Chart/1(LED_trigger)
  in1/1 -> Chart/2(count_reached)

== system gm_lab3_p9/dataplane/Avalon Data Processing/Left Channel Processing/Signal Energy Monitor/LED_Driver/LED_persistence_control7/HDL Counter ==
  in0 : Inport  OutDataTypeStr=boolean  SampleTime=1.01725260416667e-08
  Enable_out5 : EnablePort  OutDataTypeStr=boolean
  HDL Counter : hdlsllib/Sources/HDL Counter  CountType=Free running  CountInit=double(0)  CountStep=double(1)  CountMax=25  CountFromType=Initial value  CountFrom=double(0)  CountResetPort=on  CountLoadPort=off  CountEnbPort=off  CountDirPort=off  CountDataType=Unsigned  CountWordLen=15  CountFracLen=0  CountSampTime=1.01725260416667e-08
  out0 : Outport  OutDataTypeStr=fixdt(0, 15, 0)  InitialOutput=0
  wires:
  HDL Counter/1 -> out0/1
  in0/1 -> HDL Counter/1

== system gm_lab3_p9/dataplane/Avalon Data Processing/Left Channel Processing/Signal Energy Monitor/LED_Driver/LED_persistence_control/Chart/Chart ==
  LED_trigger : Inport  OutDataTypeStr=boolean  PortDimensions=1  SampleTime=1.01725260416667e-08
  count_reached : Inport  Port=2  OutDataTypeStr=boolean  PortDimensions=1  SampleTime=1.01725260416667e-08
  Chart : Stateflow chart  TreatAsAtomicUnit=on
  LED_signal : Outport  InitialOutput=0
  counter_reset : Outport  Port=2  InitialOutput=0
  wires:
  LED_trigger/1 -> Chart/1(LED_trigger)
  count_reached/1 -> Chart/2(count_reached)
  Chart/1(LED_signal) -> LED_signal/1
  Chart/2(counter_reset) -> counter_reset/1

== system gm_lab3_p9/dataplane/Avalon Data Processing/Left Channel Processing/Signal Energy Monitor/LED_Driver/LED_persistence_control1/Chart/Chart ==
  LED_trigger : Inport  OutDataTypeStr=boolean  PortDimensions=1  SampleTime=1.01725260416667e-08
  count_reached : Inport  Port=2  OutDataTypeStr=boolean  PortDimensions=1  SampleTime=1.01725260416667e-08
  Chart : Stateflow chart  TreatAsAtomicUnit=on
  LED_signal : Outport  InitialOutput=0
  counter_reset : Outport  Port=2  InitialOutput=0
  wires:
  Chart/2(counter_reset) -> counter_reset/1
  Chart/1(LED_signal) -> LED_signal/1
  count_reached/1 -> Chart/2(count_reached)
  LED_trigger/1 -> Chart/1(LED_trigger)

== system gm_lab3_p9/dataplane/Avalon Data Processing/Left Channel Processing/Signal Energy Monitor/LED_Driver/LED_persistence_control2/Chart/Chart ==
  LED_trigger : Inport  OutDataTypeStr=boolean  PortDimensions=1  SampleTime=1.01725260416667e-08
  count_reached : Inport  Port=2  OutDataTypeStr=boolean  PortDimensions=1  SampleTime=1.01725260416667e-08
  Chart : Stateflow chart  TreatAsAtomicUnit=on
  LED_signal : Outport  InitialOutput=0
  counter_reset : Outport  Port=2  InitialOutput=0
  wires:
  Chart/2(counter_reset) -> counter_reset/1
  Chart/1(LED_signal) -> LED_signal/1
  count_reached/1 -> Chart/2(count_reached)
  LED_trigger/1 -> Chart/1(LED_trigger)
